simulink model "trial"  (R2020a)
settings: Solver=VariableStepAuto  StartTime=0.0  StopTime=10.0  RelTol=1e-3
libraries: simulink x1
settings Model: Creator=graspinglab  LastModifiedBy=graspinglab

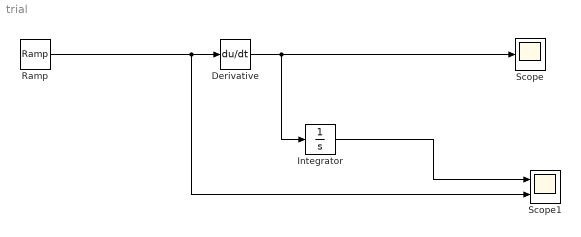
== system trial ==
  Derivative : Derivative
  Integrator : Integrator
  Ramp : simulink/Sources/Ramp  slope=1  start=0  InitialOutput=0
  Scope : Scope
  Scope1 : Scope  NumInputPorts=2
  wires:
  Ramp/1 -> Scope1/2, Derivative/1
  Derivative/1 -> Scope/1, Integrator/1
  Integrator/1 -> Scope1/1
